simulink model "analog_damped_pendulum_equation"  (R2020b)
settings: Solver=ode1be  StartTime=0.0  StopTime=30  RelTol=1e-3  AbsTol=1e-3
libraries: analogCompBlocks x13, fl_lib x2, nesl_utility x1, ee_lib x1
settings Model: DataDictionary=analogComputerData.sldd  EnableAccessToBaseWorkspace=off  OrderedModelArguments=off  Creator=roadrunner  LastModifiedBy=roadrunner
settings SolverCC: AutoScaleAbsTol=off
settings DebuggingCC: SymbolicDimsDataTypeCodeGenerationDiagnostic=none
settings SFSimCC: CustomCodeUndefinedFunction=UseInterfaceOnly
settings SimscapeCC: SimscapeLogType=all  SimscapeLogSimulationStatistics=on  SimscapeLogDataHistory=10000

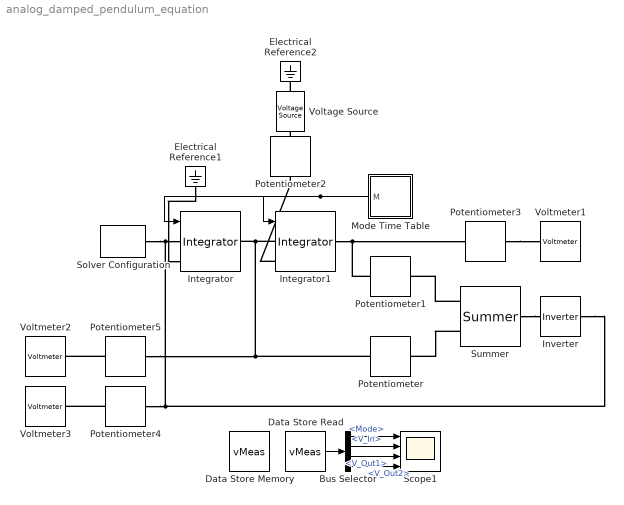
== system analog_damped_pendulum_equation ==
  Bus Selector : BusSelector  OutputSignals=Mode,V_In,V_Out1,V_Out2
  Data Store Memory : DataStoreMemory  Priority=5  DataStoreName=vMeas  ReadBeforeWriteMsg=warning  WriteAfterWriteMsg=warning  WriteAfterReadMsg=warning  ShowAdditionalParam=off  OutDataTypeStr=Bus: bus_damped_pendulum_measurements
  Data Store Read : DataStoreRead  Priority=6  DataStoreName=vMeas
  Electrical Reference1 : fl_lib/Electrical/Electrical Elements/Electrical Reference
  Electrical Reference2 : fl_lib/Electrical/Electrical Elements/Electrical Reference
  Integrator : analogCompBlocks/Integrator  capacitance=0.1  small_resistance=0.1  tau=0.1
      settings: AttributesFormatString=Integrator
  Integrator1 : analogCompBlocks/Integrator  capacitance=0.1  small_resistance=0.1  tau=0.1
      settings: AttributesFormatString=Integrator
  Inverter : analogCompBlocks/Inverter  SystemSampleTime=-1  VariantActivationTime=update diagram  Latency=0  AutoFrameSizeCalculation=off
      settings: AttributesFormatString=Inverter
  Mode Time Table : Subsystem  Priority=0  mask{DSNAME='vMeas', DSELEMENT='Mode'}
      mask prompts: DSNAME "Data Store Name"; DSELEMENT "Data Store Element"
      mask init:
      | % % Set data store name
      | % DSBLOCK = [gcb '/DataStoreWrite'];
      | % set_param(DSBLOCK,'DataStoreName',DSNAME)
      | % 
      | % % Set data store write element
      | % DSELEMENT = [DSNAME '.' DSELEMENT];
      | % set_param(DSBLOCK,'DataStoreElements',DSELEMENT)
      settings: AttributesFormatString=|
      | Mode Time
      | Table
  Potentiometer : analogCompBlocks/Potentiometer  wiper_position=0.01  max_resistance=1  gain=1
      settings: AttributesFormatString=|
      | Potentiometer
      | K/LM
  Potentiometer1 : analogCompBlocks/Potentiometer  wiper_position=0.98  max_resistance=1  gain=1
      settings: AttributesFormatString=|
      | Potentiometer
      | g/L
  Potentiometer2 : analogCompBlocks/Potentiometer  wiper_position=15*pi/180  max_resistance=0.1  gain=1
      settings: AttributesFormatString=|
      | Potentiometer
      | q0
  Potentiometer3 : analogCompBlocks/Potentiometer  wiper_position=180/pi/100  max_resistance=1  gain=100
      settings: AttributesFormatString=|
      | Potentiometer
      | rad2deg
  Potentiometer4 : analogCompBlocks/Potentiometer  wiper_position=180/pi/100  max_resistance=1  gain=100
      settings: AttributesFormatString=|
      | Potentiometer
      | rad2deg
  Potentiometer5 : analogCompBlocks/Potentiometer  wiper_position=180/pi/100  max_resistance=1  gain=100
      settings: AttributesFormatString=|
      | Potentiometer
      | rad2deg
  Scope1 : Scope  NumInputPorts=4
  Solver Configuration : nesl_utility/Solver Configuration  PhysicalDomain=network_engine_domain  SubClassName=solver  LeftPortType=input  RightPortType=generic  Tones=[]  Harmonics=[]  SimulateNoise=off  Profile=off  UseLocalSampling=off  EnableSwitchedLinearOptims=on  FrequencyDomain=off  UseCCode=off  RelTol=0.001  AbsTol=1e-06  MinStep=1e-09  ToWorkspace=off  RevertToSquareIcSolve=off  NumHomotopyIterations=100  PhasorMode=off  PhasorModeNumHarmonics=1  DoDC=off  ResidualTolerance=1e-09  UseLocalSolver=on  LocalSolverChoice=NE_BACKWARD_EULER_ADVANCER  LocalSolverSampleTime=0.01  DoFixedCost=on  MaxNonlinIter=3  MaxModeIter=2  ComputeImpulses=off  ImpulseIterations=2  LinearAlgebra=auto  EquationFormulation=NE_TIME_EF  DelaysMemoryBudget=1024  AutomaticFiltering=on  FilteringTimeConstant=0.001  PartitionStorageMethod=AS_NEEDED  PartitionMemoryBudget=1024  PartitionMethod=ROBUST
      settings: SourceProductName=Utilities
  Summer : analogCompBlocks/Summer  SystemSampleTime=-1  VariantActivationTime=update diagram  Latency=0  AutoFrameSizeCalculation=off
      settings: AttributesFormatString=Summer
  Voltage Source : ee_lib/Sources/Voltage Source  dc_voltage=1 V  ac_voltage=0 V  ac_shift=0 rad  ac_frequency=60 Hz  noise_mode=0  PSD=0 V^2/Hz  repeatability=1  auto_seed=4000182670  user_seed=0  sample_time=1e-3 s  i_specify=off  i_priority=None  i=0 A  i_nominal_specify=off  i_nominal_unit=A  i_nominal_value=1  v_specify=off  v_priority=None  v=0 V  v_nominal_specify=off  v_nominal_unit=V  v_nominal_value=1
      settings: AttributesFormatString=Constant Voltage
  Voltmeter1 : analogCompBlocks/Voltmeter  Priority=4  DSNAME='vMeas'  DSELEMENT='V_Out2'
      settings: AttributesFormatString=|
      | Voltage Sensor
      | V_Out2
  Voltmeter2 : analogCompBlocks/Voltmeter  Priority=4  DSNAME='vMeas'  DSELEMENT='V_Out1'
      settings: AttributesFormatString=|
      | Voltage Sensor
      | V_Out1
  Voltmeter3 : analogCompBlocks/Voltmeter  Priority=4  DSNAME='vMeas'  DSELEMENT='V_In'
      settings: AttributesFormatString=|
      | Voltage Sensor
      | V_In
  wires:
  Data Store Read/1 -> Bus Selector/1
  Mode Time Table/1(M) -> Integrator/1, Integrator1/1
  Bus Selector/1 -> Scope1/1  "<Mode>"
  Bus Selector/2 -> Scope1/2  "<V_In>"
  Bus Selector/3 -> Scope1/3  "<V_Out1>"
  Bus Selector/4 -> Scope1/4  "<V_Out2>"
  connections:
  Solver Configuration/RConn1 -- Inverter/RConn1 -- Potentiometer4/LConn1 -- Integrator/LConn1
  Integrator1/RConn1 -- Potentiometer3/LConn1 -- Potentiometer1/LConn1
  Electrical Reference1/LConn1 -- Integrator/LConn2
  Integrator1/LConn2 -- Potentiometer2/RConn1
  Integrator1/LConn1 -- Potentiometer5/LConn1 -- Potentiometer/LConn1 -- Integrator/RConn1
  Summer/LConn1 -- Potentiometer1/RConn1
  Summer/LConn2 -- Potentiometer/RConn1
  Voltage Source/RConn1 -- Electrical Reference2/LConn1
  Potentiometer2/LConn1 -- Voltage Source/LConn1
  Summer/RConn1 -- Inverter/LConn1
  Potentiometer3/RConn1 -- Voltmeter1/LConn1
  Potentiometer4/RConn1 -- Voltmeter3/LConn1
  Potentiometer5/RConn1 -- Voltmeter2/LConn1

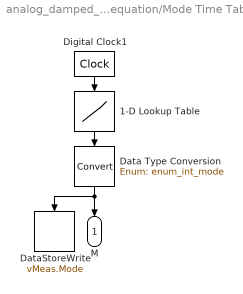
== system analog_damped_pendulum_equation/Mode Time Table ==
  1-D Lookup Table : Lookup_n-D  NumberOfTableDimensions=1  BreakpointsForDimension1=[0 5 10 20]  Table=[1 0 2 1]  InterpMethod=Flat  ExtrapMethod=Clip  InternalRulePriority=Speed  OutDataTypeStr=int32  RndMeth=Simplest  InputSameDT=on
      settings: AttributesFormatString=|
      | Integrator Mode
      | Time Table
  Data Type Conversion : DataTypeConversion  OutDataTypeStr=Enum: enum_int_mode
      settings: AttributesFormatString=|
      | Convert to
      | Mode Enum
  DataStoreWrite : DataStoreWrite  DataStoreName=vMeas  DataStoreElements=vMeas.Mode
  Digital Clock1 : DigitalClock  SampleTime=0.01
      settings: AttributesFormatString=Timer
  M : Outport
  wires:
  1-D Lookup Table/1 -> Data Type Conversion/1
  Digital Clock1/1 -> 1-D Lookup Table/1
  Data Type Conversion/1 -> DataStoreWrite/1, M/1
